simulink model "conversor_avg"  (R2024a)
settings: Solver=FixedStepAuto  StartTime=0.0  StopTime=0.01  FixedStep=0.0001  RelTol=1e-3
model workspace: external: MATLAB File Dat_DCDC_bus_batt.m (data not in the file)
undefined symbols (not defined in the file): C, L, rc, rPre, Vin
settings Model: Creator=Henrique Mesquita  LastModifiedBy=Henrique Mesquita
settings OptimizationCC: ReuseModelBlockBuffer=off
settings ModelReferenceCC: EnableParallelModelReferenceBuilds=on  ParallelModelReferenceMATLABWorkerInit=Load Top Model
settings RTWCC: GPUComputeCapability=3.5

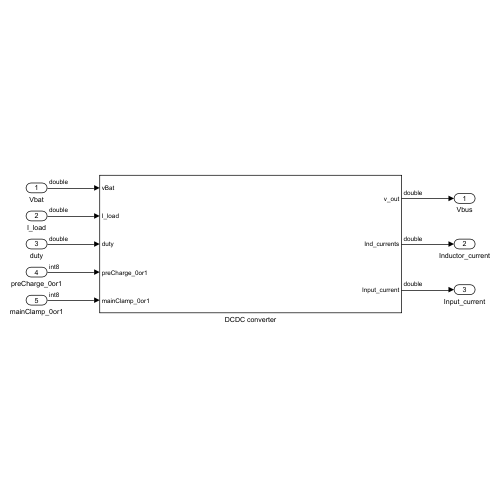
[thumbnail: Simulink's stored preview of the top-level diagram]
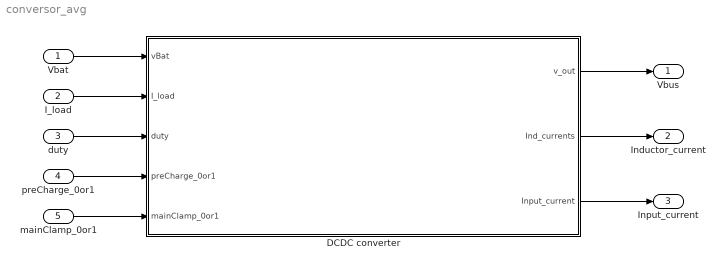
== system conversor_avg ==
  Vbat : Inport
  I_load : Inport  Port=2
  duty : Inport  Port=3
  preCharge_0or1 : Inport  Port=4  OutDataTypeStr=int8
  mainClamp_0or1 : Inport  Port=5  OutDataTypeStr=int8
  DCDC converter : Subsystem
  Vbus : Outport
  Inductor_current : Outport  Port=2
  Input_current : Outport  Port=3
  wires:
  DCDC converter/1(v_out) -> Vbus/1
  DCDC converter/2(Ind_currents) -> Inductor_current/1
  Vbat/1 -> DCDC converter/1(vBat)
  I_load/1 -> DCDC converter/2(I_load)
  duty/1 -> DCDC converter/3(duty)
  DCDC converter/3(Input_current) -> Input_current/1
  preCharge_0or1/1 -> DCDC converter/4(preCharge_0or1)
  mainClamp_0or1/1 -> DCDC converter/5(mainClamp_0or1)

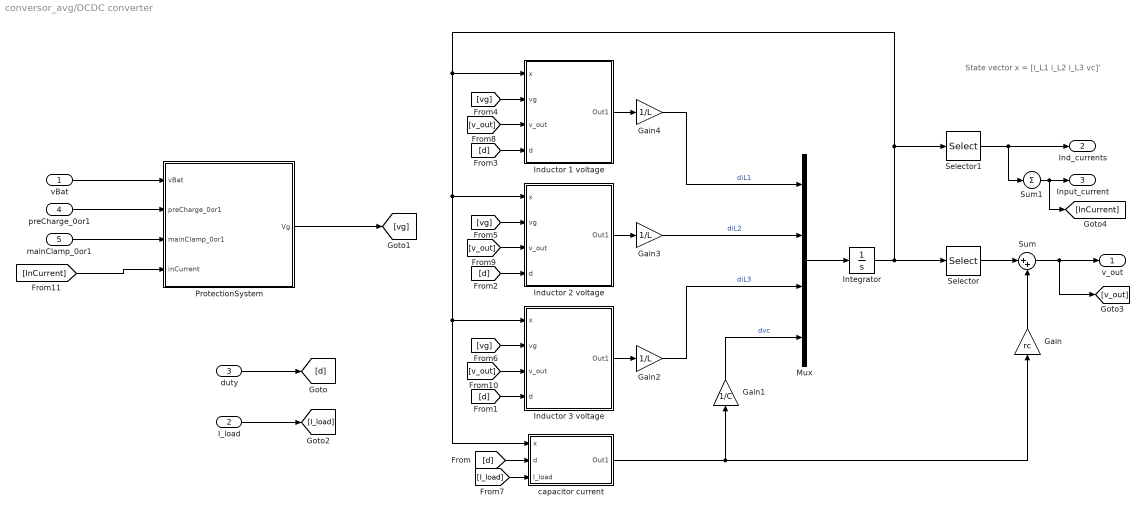
== system conversor_avg/DCDC converter ==
  note: State vector
      | x = [i_L1 i_L2 i_L3 vc]'
  vBat : Inport
  I_load : Inport  Port=2
  duty : Inport  Port=3
  preCharge_0or1 : Inport  Port=4
  mainClamp_0or1 : Inport  Port=5
  Gain : Gain  Gain=rc
  Gain1 : Gain  Gain=1/C
  Gain2 : Gain  Gain=1/L
  Gain3 : Gain  Gain=1/L
  Gain4 : Gain  Gain=1/L
  Inductor 1 voltage : Subsystem
  Inductor 2 voltage : Subsystem
  Inductor 3 voltage : Subsystem
  Integrator : Integrator  InitialCondition=[0;0;0;Vin]
  Mux : Mux
  ProtectionSystem : Subsystem
  Selector : Selector  InputPortWidth=4  IndexOptions=Index vector (dialog)  Indices=[4]  OutputSizes=1
  Selector1 : Selector  InputPortWidth=4  IndexOptions=Index vector (dialog)  Indices=[1 2 3]  OutputSizes=1
  Sum : Sum  Inputs=|++
  Sum1 : Sum  Inputs=+
  capacitor current : Subsystem
  v_out : Outport
  Ind_currents : Outport  Port=2
  Input_current : Outport  Port=3
  wires:
  duty/1 -> [d]
  Integrator/1 -> Selector/1, Selector1/1, Inductor 2 voltage/1(x), Inductor 3 voltage/1(x), capacitor current/1(x), Inductor 1 voltage/1(x)
  [d] -> capacitor current/2(d)
  Mux/1 -> Integrator/1
  Inductor 2 voltage/1(Out1) -> Gain3/1
  Inductor 3 voltage/1(Out1) -> Gain2/1
  capacitor current/1(Out1) -> Gain/1, Gain1/1
  Inductor 1 voltage/1(Out1) -> Gain4/1
  Gain1/1 -> Mux/4  "dvc"
  Gain2/1 -> Mux/3  "diL3"
  Gain3/1 -> Mux/2  "diL2"
  Gain4/1 -> Mux/1  "diL1"
  Selector/1 -> Sum/1
  Selector1/1 -> Sum1/1, Ind_currents/1
  [d] -> Inductor 1 voltage/4(d)
  [vg] -> Inductor 1 voltage/2(vg)
  I_load/1 -> [I_load]
  [I_load] -> capacitor current/3(I_load)
  Gain/1 -> Sum/2
  Sum/1 -> [v_out], v_out/1
  [v_out] -> Inductor 1 voltage/3(v_out)
  [v_out] -> Inductor 2 voltage/3(v_out)
  [vg] -> Inductor 2 voltage/2(vg)
  [d] -> Inductor 2 voltage/4(d)
  [v_out] -> Inductor 3 voltage/3(v_out)
  [vg] -> Inductor 3 voltage/2(vg)
  [d] -> Inductor 3 voltage/4(d)
  Sum1/1 -> [InCurrent], Input_current/1
  vBat/1 -> ProtectionSystem/1(vBat)
  preCharge_0or1/1 -> ProtectionSystem/2(preCharge_0or1)
  mainClamp_0or1/1 -> ProtectionSystem/3(mainClamp_0or1)
  ProtectionSystem/1(Vg) -> [vg]
  [InCurrent] -> ProtectionSystem/4(inCurrent)

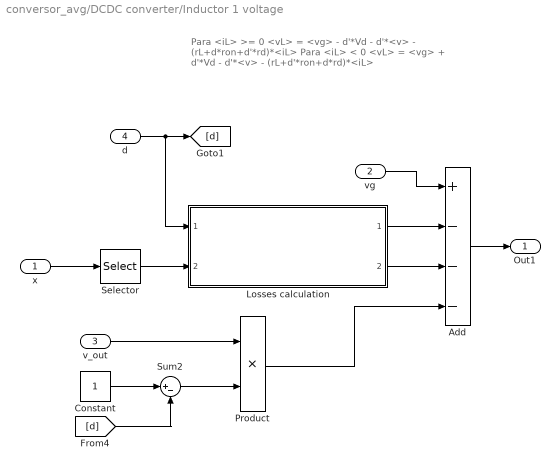
== system conversor_avg/DCDC converter/Inductor 1 voltage ==
  note: Para <iL> >= 0
      | <vL> = <vg> - d'*Vd - d'*<v> - (rL+d*ron+d'*rd)*<iL>
      | Para <iL> < 0
      | <vL> = <vg> + d'*Vd - d'*<v> - (rL+d'*ron+d*rd)*<iL>
  x : Inport
  vg : Inport  Port=2
  v_out : Inport  Port=3
  d : Inport  Port=4
  Add : Sum  Inputs=+---
  Constant : Constant
  Losses calculation : Subsystem  ReferencedSubsystem=Losses_calculation
  Product : Product
  Selector : Selector  InputPortWidth=4  IndexOptions=Index vector (dialog)  Indices=[1]  OutputSizes=1
  Sum2 : Sum  Inputs=|+-
  Out1 : Outport
  wires:
  vg/1 -> Add/1
  Product/1 -> Add/4
  x/1 -> Selector/1
  d/1 -> Losses calculation/1, [d]
  v_out/1 -> Product/1
  Selector/1 -> Losses calculation/2
  Add/1 -> Out1/1
  Constant/1 -> Sum2/1
  Sum2/1 -> Product/2
  [d] -> Sum2/2
  Losses calculation/1 -> Add/2
  Losses calculation/2 -> Add/3

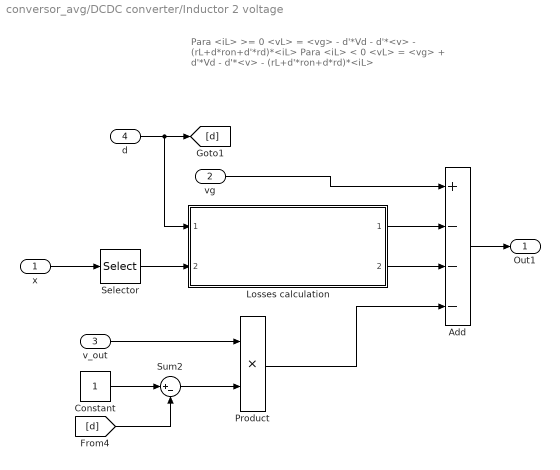
== system conversor_avg/DCDC converter/Inductor 2 voltage ==
  note: Para <iL> >= 0
      | <vL> = <vg> - d'*Vd - d'*<v> - (rL+d*ron+d'*rd)*<iL>
      | Para <iL> < 0
      | <vL> = <vg> + d'*Vd - d'*<v> - (rL+d'*ron+d*rd)*<iL>
  x : Inport
  vg : Inport  Port=2
  v_out : Inport  Port=3
  d : Inport  Port=4
  Add : Sum  Inputs=+---
  Constant : Constant
  Losses calculation : Subsystem  ReferencedSubsystem=Losses_calculation
  Product : Product
  Selector : Selector  InputPortWidth=4  IndexOptions=Index vector (dialog)  Indices=[2]  OutputSizes=1
  Sum2 : Sum  Inputs=|+-
  Out1 : Outport
  wires:
  vg/1 -> Add/1
  Product/1 -> Add/4
  x/1 -> Selector/1
  d/1 -> Losses calculation/1, [d]
  v_out/1 -> Product/1
  Selector/1 -> Losses calculation/2
  Add/1 -> Out1/1
  Constant/1 -> Sum2/1
  Sum2/1 -> Product/2
  [d] -> Sum2/2
  Losses calculation/1 -> Add/2
  Losses calculation/2 -> Add/3

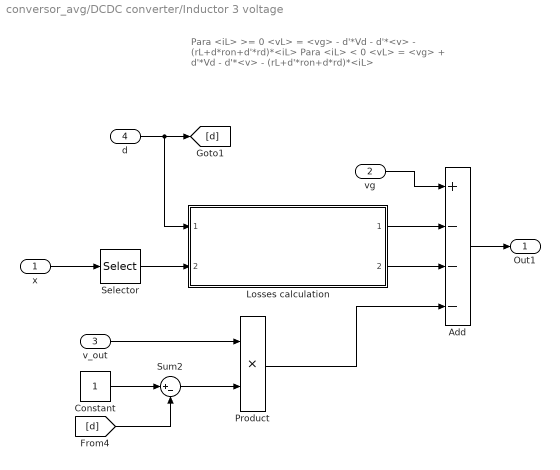
== system conversor_avg/DCDC converter/Inductor 3 voltage ==
  note: Para <iL> >= 0
      | <vL> = <vg> - d'*Vd - d'*<v> - (rL+d*ron+d'*rd)*<iL>
      | Para <iL> < 0
      | <vL> = <vg> + d'*Vd - d'*<v> - (rL+d'*ron+d*rd)*<iL>
  x : Inport
  vg : Inport  Port=2
  v_out : Inport  Port=3
  d : Inport  Port=4
  Add : Sum  Inputs=+---
  Constant : Constant
  Losses calculation : Subsystem  ReferencedSubsystem=Losses_calculation
  Product : Product
  Selector : Selector  InputPortWidth=4  IndexOptions=Index vector (dialog)  Indices=[3]  OutputSizes=1
  Sum2 : Sum  Inputs=|+-
  Out1 : Outport
  wires:
  vg/1 -> Add/1
  Product/1 -> Add/4
  x/1 -> Selector/1
  d/1 -> Losses calculation/1, [d]
  v_out/1 -> Product/1
  Selector/1 -> Losses calculation/2
  Add/1 -> Out1/1
  Constant/1 -> Sum2/1
  Sum2/1 -> Product/2
  [d] -> Sum2/2
  Losses calculation/1 -> Add/2
  Losses calculation/2 -> Add/3

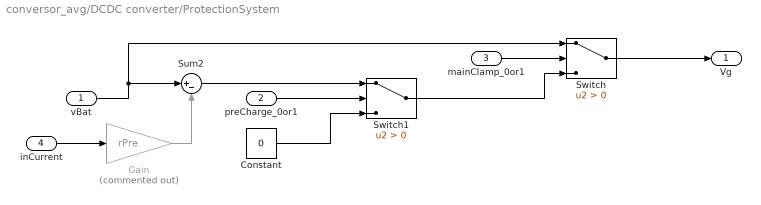
== system conversor_avg/DCDC converter/ProtectionSystem ==
  vBat : Inport
  preCharge_0or1 : Inport  Port=2
  mainClamp_0or1 : Inport  Port=3
  inCurrent : Inport  Port=4
  Constant : Constant  Value=0
  Gain : Gain  Commented=on  Gain=rPre
  Sum2 : Sum  Inputs=|+-
  Switch : Switch  Criteria=u2 > Threshold  SaturateOnIntegerOverflow=off  InputSameDT=off
  Switch1 : Switch  Criteria=u2 > Threshold  SaturateOnIntegerOverflow=off  InputSameDT=off
  Vg : Outport
  wires:
  inCurrent/1 -> Gain/1
  preCharge_0or1/1 -> Switch1/2
  Gain/1 -> Sum2/2
  mainClamp_0or1/1 -> Switch/2
  vBat/1 -> Switch/1, Sum2/1
  Switch/1 -> Vg/1
  Constant/1 -> Switch1/3
  Switch1/1 -> Switch/3
  Sum2/1 -> Switch1/1

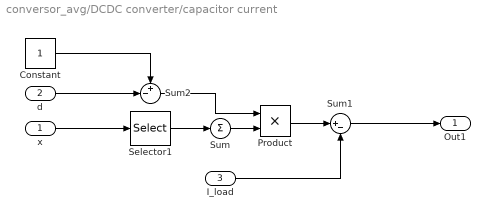
== system conversor_avg/DCDC converter/capacitor current ==
  x : Inport
  d : Inport  Port=2
  I_load : Inport  Port=3
  Constant : Constant
  Product : Product
  Selector1 : Selector  InputPortWidth=4  IndexOptions=Index vector (dialog)  Indices=[1 2 3]  OutputSizes=1
  Sum : Sum  Inputs=+
  Sum1 : Sum  Inputs=|+-
  Sum2 : Sum  Inputs=+-|
  Out1 : Outport
  wires:
  Selector1/1 -> Sum/1
  x/1 -> Selector1/1
  I_load/1 -> Sum1/2
  Sum1/1 -> Out1/1
  Sum/1 -> Product/2
  Sum2/1 -> Product/1
  Product/1 -> Sum1/1
  d/1 -> Sum2/2
  Constant/1 -> Sum2/1
